simulink model "lab_2"  (R2015a)
settings: Solver=ode45  StartTime=0.0  StopTime=10.0  RelTol=1e-3
values from neighbouring files (symbols this model uses):
  A = [1.37189711143 1 0 0 0 0 0.796247030428 0 1 0 0 0 ... (36 elements, 6x6)]    [matrizes.mat]
  B = [1 0 0 0 0 0]    [matrizes.mat]
  C = [0.176432501593 -0.307260665336 -0.097075632123 0.119078500307 -0.365349527089 0]    [matrizes.mat]
  D = 0    [matrizes.mat]
  K = [0.152892335406 -0.0494306399458 -0.17992491845 0.0741519455973 0.109452261993 -0.0633139239932]    [matrizes.mat]
  M = [-4.02099236255 -3.77131879733 -2.84355374965 -1.32107837653 -1.17257932747 0.607476554194]    [matrizes.mat]
  Nbar = -2.20135488168    [matrizes.mat]    (also in script_lab2.m = Nu+K*Nx)
settings Model: Creator=Alunos  LastModifiedBy=Alunos

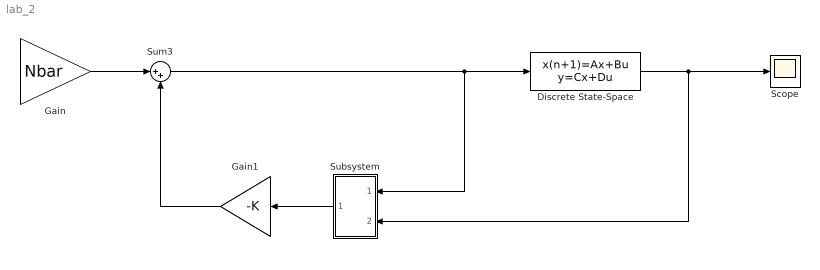
== system lab_2 ==
  Discrete State-Space : DiscreteStateSpace  A=A  B=B  C=C  D=D  SampleTime=0.02
  Gain : Gain  Gain=Nbar
  Gain1 : Gain  Gain=-K
  Scope : Scope
      settings: SaveName=y_final
  Subsystem : Subsystem
  Sum3 : Sum  Inputs=|++
  wires:
  Sum3/1 -> Subsystem/1(In1), Discrete State-Space/1
  Gain/1 -> Sum3/1
  Gain1/1 -> Sum3/2
  Discrete State-Space/1 -> Scope/1, Subsystem/2(In2)
  Subsystem/1(Out1) -> Gain1/1

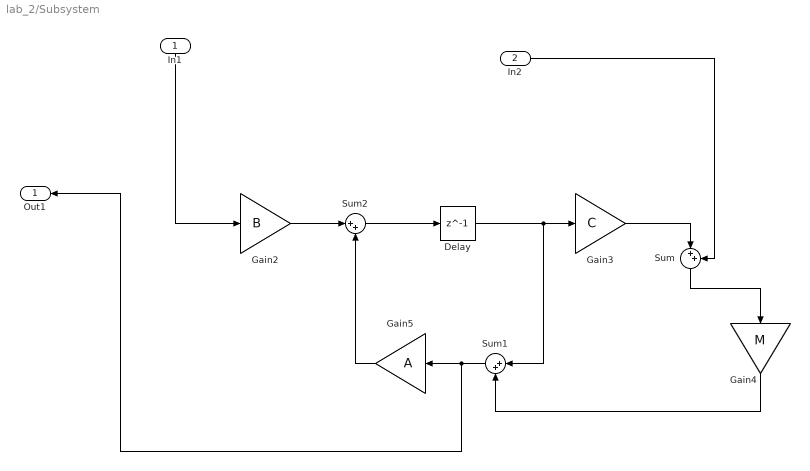
== system lab_2/Subsystem ==
  In1 : Inport
  In2 : Inport  Port=2
  Delay : Delay  DelayLength=1  InitialCondition=0
  Gain2 : Gain  Gain=B
  Gain3 : Gain  Gain=C
  Gain4 : Gain  Gain=M
  Gain5 : Gain  Gain=A
  Sum : Sum  Inputs=|++
  Sum1 : Sum  Inputs=|++
  Sum2 : Sum  Inputs=|++
  Out1 : Outport
  wires:
  Gain3/1 -> Sum/1
  In1/1 -> Gain2/1
  Gain4/1 -> Sum1/2
  Sum/1 -> Gain4/1
  Gain5/1 -> Sum2/2
  Sum1/1 -> Out1/1, Gain5/1
  In2/1 -> Sum/2
  Sum2/1 -> Delay/1
  Delay/1 -> Sum1/1, Gain3/1
  Gain2/1 -> Sum2/1
